simulink library "vmc"  (R2021b)
settings: Solver=VariableStepAuto  StartTime=0.0  StopTime=10.0  RelTol=1e-3
undefined symbols (not defined in the file): AVMC_ACCDeltaTqGradeGn_X_deg, AVMC_ACCDeltaTqIGain4OVRD_X_kph, AVMC_ACCDeltaTqIGain4OVRD_Y_mps2, AVMC_ACCDeltaTqIGain_X_kph, AVMC_ACCDeltaTqIGain_Y_mps2, AVMC_ACCDeltaTqPGain_X_kph, AVMC_ACCDeltaTqPGain_Y_kph, AVMC_ACCGradeofst_X_G, AVMC_ACCGradeofst_Y_pct, AVMC_ACCLoSpdTqLoLim4JP_X_kph, AVMC_ACCLoSpdTqLoLim4JP_Y_deg, AVMC_ACCLoSpdTqLowerLim_X_kph, AVMC_ACCLoSpdTqLowerLim_Y_deg, AVMC_ACCReqAccelGain_X_mps2, AVMC_ACCReqAccelGain_Y_enum, AVMC_ADSPosGFBDeltaTq_X_kph, AVMC_ADSPosGFBDeltaTq_Y_mps2, AVMC_AggressJerkPCT4AT_X_kph, AVMC_AggressJerkPCT_X_kph, AVMC_AggressLimitPCT4AT_X_kph, AVMC_AggressLimitPCT_X_kph, AVMC_DECGradeofst_X_G, AVMC_DECGradeofst_Y_pct, AVMC_DISCDeltaTqIGain_X_kph, AVMC_DISCDeltaTqIGain_Y_mps2, AVMC_DISCDeltaTqPGain_X_kph, AVMC_DISCDeltaTqPGain_Y_kph, AVMC_EPSForceSelect_X_enum, AVMC_EPSForceSelect_Y_enum, AVMC_EPSForceSelectD21_X_enum, AVMC_EPSForceSelectD21_Y_enum, AVMC_ESCRegenOut_X_kph, AVMC_ESCRegenOut_Y_Deg, AVMC_ESCRegenOutEnSpd_X_Deg, AVMC_EstPitchSlopeTs_X_kph, AVMC_GradeCompFlt_X_kph, AVMC_GyroYBandLo_X_Gps, AVMC_HoldResTq_X_kph, AVMC_ISOAccLimit_X_mps, AVMC_ISODecLimit_X_mps, AVMC_ISOJerk_X_mps, AVMC_LatESCRegenOut_X_kph, AVMC_LatESCRegenOut_Y_Deg, AVMC_LongAccDeadZone_X_kph, AVMC_LongAccFiltTsforP2_X_Gps, AVMC_MCPresBaseTq_X_bar, AVMC_MSAPedalOvrd_X_kph, AVMC_MSASpdBand_X_kph, AVMC_MSATqDownEndTq_X_kph, AVMC_MSATqDownTime_X_kph, AVMC_NegZCHoldTq_X_kph, AVMC_OPDDisSlideRate_X_Deg, AVMC_OVRD2ActSR2FCMCMD_X_mps2, AVMC_PedalTqRWhlRatio_X_Nm, AVMC_PedalTqRWhlRatio_Y_gps, AVMC_PedalTqRWhlSlipGain_X_rat, AVMC_PedalTqRWhlSlipGain_Y_kph, AVMC_PedalTqRWhSTRGGain_X_deg, AVMC_PedalTqRWhSTRGGain_Y_kph, AVMC_PosZCHoldTq_X_kph ... (+593)
libraries: hcu_lib x143, simulink x96, tqr x4, $bdroot x1, simulink_extras x1
(part 15 of 17)

== system vmc/VMC/VMC/Long Acceleration Calculation/Estimate Slope1/SR_Latch1 ==
  set : Inport
  reset : Inport  Port=2
  Data Type Conversion : DataTypeConversion  OutDataTypeStr=boolean
  Logical Operator : Logic  AllPortsSameDT=off  OutDataTypeStr=boolean
  Logical Operator1 : Logic  Operator=NOT  AllPortsSameDT=off  OutDataTypeStr=boolean
  Switch1 : Switch  Criteria=u2 ~= 0  Threshold=0.5
      settings: AttributesFormatString=<Criteria=%<Criteria>>
  Switch2 : Switch  Criteria=u2 ~= 0  Threshold=0.5
      settings: AttributesFormatString=<Criteria=%<Criteria>>
  Unit Delay : UnitDelay  SampleTime=-1  HasFrameUpgradeWarning=on
  latched : Outport
  wires:
  Data Type Conversion/1 -> Unit Delay/1, latched/1
  Switch1/1 -> Data Type Conversion/1
  set/1 -> Switch1/1, Logical Operator/1
  reset/1 -> Switch2/2, Logical Operator1/1
  Unit Delay/1 -> Switch2/3
  Switch2/1 -> Switch1/3
  Logical Operator/1 -> Switch1/2
  Logical Operator1/1 -> Logical Operator/2, Switch2/1

== system vmc/VMC/VMC/Long Acceleration Calculation/Estimate Slope1/SR_Latch2 ==
  set : Inport
  reset : Inport  Port=2
  Data Type Conversion : DataTypeConversion  OutDataTypeStr=boolean
  Logical Operator : Logic  AllPortsSameDT=off  OutDataTypeStr=boolean
  Logical Operator1 : Logic  Operator=NOT  AllPortsSameDT=off  OutDataTypeStr=boolean
  Switch1 : Switch  Criteria=u2 ~= 0  Threshold=0.5
      settings: AttributesFormatString=<Criteria=%<Criteria>>
  Switch2 : Switch  Criteria=u2 ~= 0  Threshold=0.5
      settings: AttributesFormatString=<Criteria=%<Criteria>>
  Unit Delay : UnitDelay  SampleTime=-1  HasFrameUpgradeWarning=on
  latched : Outport
  wires:
  Logical Operator1/1 -> Switch2/1, Logical Operator/2
  Logical Operator/1 -> Switch1/2
  Switch2/1 -> Switch1/3
  Unit Delay/1 -> Switch2/3
  reset/1 -> Logical Operator1/1, Switch2/2
  set/1 -> Logical Operator/1, Switch1/1
  Switch1/1 -> Data Type Conversion/1
  Data Type Conversion/1 -> latched/1, Unit Delay/1

== system vmc/VMC/VMC/Long Acceleration Calculation/Estimate Slope1/SR_Latch3 ==
  set : Inport
  reset : Inport  Port=2
  Data Type Conversion : DataTypeConversion  OutDataTypeStr=boolean
  Logical Operator : Logic  AllPortsSameDT=off  OutDataTypeStr=boolean
  Logical Operator1 : Logic  Operator=NOT  AllPortsSameDT=off  OutDataTypeStr=boolean
  Switch1 : Switch  Criteria=u2 ~= 0  Threshold=0.5
      settings: AttributesFormatString=<Criteria=%<Criteria>>
  Switch2 : Switch  Criteria=u2 ~= 0  Threshold=0.5
      settings: AttributesFormatString=<Criteria=%<Criteria>>
  Unit Delay : UnitDelay  SampleTime=-1  HasFrameUpgradeWarning=on
  latched : Outport
  wires:
  Logical Operator1/1 -> Switch2/1, Logical Operator/2
  Logical Operator/1 -> Switch1/2
  Switch2/1 -> Switch1/3
  Unit Delay/1 -> Switch2/3
  reset/1 -> Logical Operator1/1, Switch2/2
  set/1 -> Logical Operator/1, Switch1/1
  Switch1/1 -> Data Type Conversion/1
  Data Type Conversion/1 -> latched/1, Unit Delay/1

== system vmc/VMC/VMC/Long Acceleration Calculation/Estimate Slope1/SR_Latch6 ==
  set : Inport
  reset : Inport  Port=2
  Data Type Conversion : DataTypeConversion  OutDataTypeStr=boolean
  Logical Operator : Logic  AllPortsSameDT=off  OutDataTypeStr=boolean
  Logical Operator1 : Logic  Operator=NOT  AllPortsSameDT=off  OutDataTypeStr=boolean
  Switch1 : Switch  Criteria=u2 ~= 0  Threshold=0.5
      settings: AttributesFormatString=<Criteria=%<Criteria>>
  Switch2 : Switch  Criteria=u2 ~= 0  Threshold=0.5
      settings: AttributesFormatString=<Criteria=%<Criteria>>
  Unit Delay : UnitDelay  SampleTime=-1  HasFrameUpgradeWarning=on
  latched : Outport
  wires:
  Logical Operator1/1 -> Switch2/1, Logical Operator/2
  Logical Operator/1 -> Switch1/2
  Switch2/1 -> Switch1/3
  Unit Delay/1 -> Switch2/3
  reset/1 -> Logical Operator1/1, Switch2/2
  set/1 -> Logical Operator/1, Switch1/1
  Switch1/1 -> Data Type Conversion/1
  Data Type Conversion/1 -> latched/1, Unit Delay/1

== system vmc/VMC/VMC/Long Acceleration Calculation/Estimate Slope1/Triggered Subsystem ==
  In1 : Inport
  Trigger : TriggerPort  VariantControl=(inherit)
  Out1 : Outport
  wires:
  In1/1 -> Out1/1

== system vmc/VMC/VMC/MSA function/MSADemandTorqueCalculation/Triggered Subsystem ==
  In1 : Inport
  Trigger : TriggerPort  VariantControl=(inherit)
  Out1 : Outport
  wires:
  In1/1 -> Out1/1

== system vmc/VMC/VMC/MSA function/MSATorqueSourceDetermination/Triggered Subsystem2 ==
  In1 : Inport
  Trigger : TriggerPort  VariantControl=(inherit)
  Out1 : Outport
  wires:
  In1/1 -> Out1/1

== system vmc/VMC/VMC/SPD2ACC/Required_Acceleration/Triggered Subsystem ==
  In1 : Inport
  In2 : Inport  Port=2
  Trigger : TriggerPort  VariantControl=(inherit)
  Add29 : Sum  Inputs=+-
  Constant216 : Constant  Value=KVMC_ReqBrkInDecSRTime_s
  Divide : Product  Inputs=*/
  Out1 : Outport
  wires:
  In1/1 -> Add29/2
  In2/1 -> Add29/1
  Add29/1 -> Divide/1
  Constant216/1 -> Divide/2
  Divide/1 -> Out1/1

== system vmc/VMC/VMC/SPD2ACC/Required_Acceleration/Triggered Subsystem4 ==
  In1 : Inport
  Trigger : TriggerPort  VariantControl=(inherit)
  Out1 : Outport
  wires:
  In1/1 -> Out1/1

== system vmc/VMC/VMC/SPD2ACC/Required_Acceleration/Triggered Subsystem6 ==
  In1 : Inport
  In2 : Inport  Port=2
  In3 : Inport  Port=3
  Trigger : TriggerPort  VariantControl=(inherit)
  Out1 : Outport
  Out2 : Outport  Port=2
  Out3 : Outport  Port=3
  wires:
  In3/1 -> Out3/1
  In2/1 -> Out2/1
  In1/1 -> Out1/1

== system vmc/VMC/VMC/SPD2ACC/Required_Acceleration/Triggered Subsystem7 ==
  In1 : Inport
  Trigger : TriggerPort  VariantControl=(inherit)
  Out1 : Outport
  wires:
  In1/1 -> Out1/1

== system vmc/VMC/VMC/SafetyControl/LongAccel_EstSlope_FrontRearSlipSpd/Estimate Slope ==
  VINP_LongAccel_Gps : Inport
  VVMC_VehicleSpeed_kph : Inport  Port=2
  VINP_GRADE_deg : Inport  Port=3
  task_time_s : Inport  Port=4
  Add : Sum  Inputs=+-
  Asin : Trigonometry  Operator=asin
  Constant : Constant  Tag=struct('comment',struct('text','','placement',1),'output',struct('width',1,'name','$S_$B','unit','','type','Int16','offset',0,'max',NaN,'min',NaN,'freeze',1,'lsb',1,'arb',0,'class','default','address','','description','','value','0','tolerance',1,'show',0),'date',731450.689904282)  Value=ZERO_FLOAT  OutDataTypeStr=single
  Constant1 : Constant  Value=KVMC_EstSlopeLongAccelTs_c
  Constant2 : Constant  Value=KVMC_EstSlopeVehSpdTs_c
  Constant28 : Constant  Value=MINUSONE_FLOAT
  Constant29 : Constant  Value=ONE_FLOAT
  Constant3 : Constant  Value=KVMC_EstSlopeTs_c
  Constant4 : Constant  Value=KVMC_EstSlopeSW_flg
  Constant5 : Constant  Tag=struct('comment',struct('text','','placement',1),'output',struct('width',1,'name','$S_$B','unit','','type','Int16','offset',0,'max',NaN,'min',NaN,'freeze',1,'lsb',1,'arb',0,'class','default','address','','description','','value','2','tolerance',1,'show',0),'date',731450.690075)  Value=TRUE
  FirstOrderFilter : hcu_lib/Basic_Blocks/FirstOrderFilter
  FirstOrderFilter1 : hcu_lib/Basic_Blocks/FirstOrderFilter
  FirstOrderFilter2 : hcu_lib/Basic_Blocks/FirstOrderFilter
  Gain : Gain  Gain=KPH2MPS
  Gain1 : Gain  Gain=1/GRAVITY_G
  Gain2 : Gain  Gain=RAD2DEG
  Product : Product  Tag=struct('comment',struct('text','','placement',1),'logdata',struct('maxnumvals',inf,'plotchannels',[],'stepsize',0,'downsampling',1,'loggingmode',3,'channels',1),'output',struct('width',1,'name','$S_$B','unit','','type','Int32Bin15','offset',0,'max',65535,'min',-65536,'freeze',1,'lsb',2^-15,'arb',0,'class','default','address','','description','','autoscalingmode',1,'lowerheadroom',1,'upperheadroom',1,'headroomunit','bit','checkmin',0,'checkmax',0,'show',0),'inputs','*/','exceptionhandling',1,'date',731458.438505301)  Inputs=*/  InputSameDT=on  RndMeth=Zero  SaturateOnIntegerOverflow=on  OutDataTypeStr=Inherit: Same as first input
  Saturation Dynamic3 : simulink/Discontinuities/Saturation Dynamic  OutMin=[]  OutMax=[]  OutDataTypeStr=Inherit: Same as second input  OutDataType=fixdt(1, 16)  OutScaling=2^-10  DoSatur=off
  Sum : Sum  Tag=struct('comment',struct('text','','placement',1),'logdata',struct('maxnumvals',inf,'plotchannels',[],'stepsize',0,'downsampling',1,'loggingmode',3,'channels',1),'output',struct('width',1,'name','$S_$B','unit','','type','Int32Bin15','offset',0,'max',65535,'min',-65536,'freeze',1,'lsb',2^-15,'arb',0,'class','default','address','','description','','autoscalingmode',1,'lowerheadroom',1,'upperheadroom',1,'headroomunit','bit','checkmin',0,'checkmax',0,'show',0),'inputs','+-','date',731450.688943275)  Inputs=+-  InputSameDT=on  SaturateOnIntegerOverflow=on  OutDataTypeStr=Inherit: Same as first input
  Switch : Switch  Criteria=u2 > Threshold
  Switch1 : Switch  Tag=struct('comment',struct('text','','placement',1),'logdata',struct('maxnumvals',inf,'plotchannels',[],'stepsize',0,'downsampling',1,'loggingmode',3,'channels',1),'output',struct('width',1,'name','$S_$B','unit','','type','Int32Bin15','offset',0,'max',65535,'min',-65536,'freeze',1,'lsb',2^-15,'arb',0,'class','default','address','','description','','autoscalingmode',1,'lowerheadroom',1,'upperheadroom',1,'headroomunit','bit','checkmin',0,'checkmax',0,'show',0),'threshold',struct('width',1,'name','$S_$B_threshold','unit','','type','Int16','offset',0,'max',NaN,'min',NaN,'freeze',1,'lsb',1,'arb',0,'class','default','address','','description','','value','1','scalar',0),'date',731458.438569977)  Criteria=u2 > Threshold  SaturateOnIntegerOverflow=on  InputSameDT=on
  UnitDelay1 : UnitDelay  Tag=struct('comment',struct('text','','placement',1),'logdata',struct('maxnumvals',inf,'plotchannels',[],'stepsize',0,'downsampling',1,'loggingmode',3,'channels',1),'output',struct('width',1,'name','$S_$B','unit','','type','Int32Bin15','offset',0,'max',65535,'min',-65536,'freeze',1,'lsb',2^-15,'arb',0,'class','default','address','','description','','autoscalingmode',1,'lowerheadroom',1,'upperheadroom',1,'headroomunit','bit','checkmin',0,'checkmax',0,'show',0,'initial','0'),'state',0,'dt','-1','date',731450.687911019)  SampleTime=-1  HasFrameUpgradeWarning=on
  UnitDelay2 : UnitDelay  Tag=struct('comment',struct('text','','placement',1),'logdata',struct('maxnumvals',inf,'plotchannels',[],'stepsize',0,'downsampling',1,'loggingmode',3,'channels',1),'output',struct('width',1,'name','$S_$B','unit','','type','UInt8','offset',0,'max',255,'min',0,'freeze',1,'lsb',1,'arb',0,'class','default','address','','description','','autoscalingmode',1,'lowerheadroom',1,'upperheadroom',1,'headroomunit','bit','checkmin',0,'checkmax',0,'show',0,'initial','0'),'state',0,'dt','-1','date',731450.690382801)  InitialCondition=FALSE  SampleTime=-1  StateName=first_pass  HasFrameUpgradeWarning=on
  VVMC_EstSlopeCal_Deg : Outport
  wires:
  VINP_GRADE_deg/1 -> Switch/3
  Constant4/1 -> Switch/2
  [task_time_s] -> FirstOrderFilter1/2
  Constant2/1 -> FirstOrderFilter1/3
  Constant3/1 -> FirstOrderFilter2/3
  [task_time_s] -> FirstOrderFilter2/2
  Constant1/1 -> FirstOrderFilter/3
  [task_time_s] -> FirstOrderFilter/2
  Switch/1 -> VVMC_EstSlopeCal_Deg/1  "VVMC_EstSlopeCal_Deg"
  FirstOrderFilter2/1 -> Switch/1
  Gain2/1 -> FirstOrderFilter2/1
  Asin/1 -> Gain2/1
  Product/1 -> Gain1/1
  FirstOrderFilter1/1 -> Gain/1
  FirstOrderFilter/1 -> Add/1
  Add/1 -> Saturation Dynamic3/2  "sum"
  Gain1/1 -> Add/2
  VINP_LongAccel_Gps/1 -> FirstOrderFilter/1
  VVMC_VehicleSpeed_kph/1 -> FirstOrderFilter1/1
  task_time_s/1 -> [task_time_s]
  Constant/1 -> Switch1/3
  UnitDelay2/1 -> Switch1/2
  Constant5/1 -> UnitDelay2/1
  [task_time_s] -> Product/2
  UnitDelay1/1 -> Sum/2
  Gain/1 -> Sum/1, UnitDelay1/1
  Sum/1 -> Switch1/1
  Switch1/1 -> Product/1
  Constant28/1 -> Saturation Dynamic3/3
  Constant29/1 -> Saturation Dynamic3/1
  Saturation Dynamic3/1 -> Asin/1

== system vmc/VMC/VMC/SafetyControl/SafetyControlJudgement/FrontRearSlipRatio ==
  VVMC_LFWhlSpeedRollAve_kph : Inport
  VVMC_RFWhlSpeedRollAve_kph : Inport  Port=2
  VVMC_LRWhlSpeedRollAve_kph : Inport  Port=3
  VVMC_RRWhlSpeedRollAve_kph : Inport  Port=4
  VINP_LFRawWhlSpeedV_flg : Inport  Port=5
  VINP_RFRawWhlSpeedV_flg : Inport  Port=6
  VINP_LRRawWhlSpeedV_flg : Inport  Port=7
  VINP_RRRawWhlSpeedV_flg : Inport  Port=8
  Constant : Constant  Value=KVMC_FrontRearSlipRatioTHR_kph
  Constant1 : Constant  Value=TRUE
  Constant2 : Constant  Value=FALSE
  Constant3 : Constant  Value=TWO_FLOAT
  Constant4 : Constant  Value=ZERO_FLOAT
  FrontRearSlipRatioJudgement : Stateflow chart  TreatAsAtomicUnit=on
  "VVMC_FrontRearSlipRatioCtrl_flg " : Outport
  wires:
  VVMC_LFWhlSpeedRollAve_kph/1 -> [VVMC_LFWhlSpeedRollAve_kph]
  VVMC_RFWhlSpeedRollAve_kph/1 -> [VVMC_RFWhlSpeedRollAve_kph]
  VVMC_LRWhlSpeedRollAve_kph/1 -> [VVMC_LRWhlSpeedRollAve_kph]
  VVMC_RRWhlSpeedRollAve_kph/1 -> [VVMC_RRWhlSpeedRollAve_kph]
  VINP_LFRawWhlSpeedV_flg/1 -> [VINP_LFRawWhlSpeedV_flg]
  VINP_RFRawWhlSpeedV_flg/1 -> [VINP_RFRawWhlSpeedV_flg]
  VINP_LRRawWhlSpeedV_flg/1 -> [VINP_LRRawWhlSpeedV_flg]
  VINP_RRRawWhlSpeedV_flg/1 -> [VINP_RRRawWhlSpeedV_flg]
  [VINP_LRRawWhlSpeedV_flg] -> FrontRearSlipRatioJudgement/7(VINP_LRRawWhlSpeedV_flg)
  [VINP_LFRawWhlSpeedV_flg] -> FrontRearSlipRatioJudgement/5(VINP_LFRawWhlSpeedV_flg)
  [VVMC_LRWhlSpeedRollAve_kph] -> FrontRearSlipRatioJudgement/3(VVMC_LRWhlSpeedRollAve_kph)
  [VINP_RFRawWhlSpeedV_flg] -> FrontRearSlipRatioJudgement/6(VINP_RFRawWhlSpeedV_flg)
  [VVMC_LFWhlSpeedRollAve_kph] -> FrontRearSlipRatioJudgement/1(VVMC_LFWhlSpeedRollAve_kph)
  [VVMC_RFWhlSpeedRollAve_kph] -> FrontRearSlipRatioJudgement/2(VVMC_RFWhlSpeedRollAve_kph)
  [VVMC_RRWhlSpeedRollAve_kph] -> FrontRearSlipRatioJudgement/4(VVMC_RRWhlSpeedRollAve_kph)
  [VINP_RRRawWhlSpeedV_flg] -> FrontRearSlipRatioJudgement/8(VINP_RRRawWhlSpeedV_flg)
  Constant/1 -> FrontRearSlipRatioJudgement/9(KVMC_FrontRearSlipRatioTHR_kph)
  Constant1/1 -> FrontRearSlipRatioJudgement/10(TRUE)
  FrontRearSlipRatioJudgement/1(VVMC_FrontRearSlipRatioCtrl_flg) -> [VVMC_FrontRearSlipRatioCtrl_flg]
  [VVMC_FrontRearSlipRatioCtrl_flg] -> "VVMC_FrontRearSlipRatioCtrl_flg "/1
  Constant2/1 -> FrontRearSlipRatioJudgement/11(FALSE)
  Constant3/1 -> FrontRearSlipRatioJudgement/12(TWO_FLOAT)
  Constant4/1 -> FrontRearSlipRatioJudgement/13(ZERO_FLOAT)

== system vmc/VMC/VMC/SafetyControl/SafetyControlJudgement/LateralAccelerationControl ==
  VVMC_LatAccRollAve_Gps : Inport
  VINP_LatAccelV_flg : Inport  Port=2
  Abs : Abs
  Constant : Constant  Value=KVMC_LatAccCtrlTHR_Gps
  Logical Operator : Logic  Operator=OR  AllPortsSameDT=off  OutDataTypeStr=boolean
  Relational Operator : RelationalOperator  OutDataTypeStr=boolean  RndMeth=Simplest
  VVMC_LatAccCtrl_flg : Outport
  wires:
  VVMC_LatAccRollAve_Gps/1 -> [VVMC_LatAccRollAve_Gps]
  VINP_LatAccelV_flg/1 -> [VINP_LatAccelV_flg]
  [VVMC_LatAccCtrl_flg] -> VVMC_LatAccCtrl_flg/1
  [VVMC_LatAccRollAve_Gps] -> Abs/1
  Constant/1 -> Relational Operator/2
  Relational Operator/1 -> Logical Operator/1
  [VINP_LatAccelV_flg] -> Logical Operator/2
  Logical Operator/1 -> [VVMC_LatAccCtrl_flg]  "VVMC_LatAccCtrl_flg"
  Abs/1 -> Relational Operator/1

== system vmc/VMC/VMC/SafetyControl/SafetyControlJudgement/RearWheelSlipRatio ==
  VVMC_LRWhlSpeedRollAve_kph : Inport
  VVMC_RRWhlSpeedRollAve_kph : Inport  Port=2
  VINP_LRRawWhlSpeedV_flg : Inport  Port=3
  VINP_RRRawWhlSpeedV_flg : Inport  Port=4
  Constant : Constant  Value=KVMC_RearWhlSlipRatioTHR_kph
  Constant1 : Constant  Value=TRUE
  Constant2 : Constant  Value=FALSE
  FrontRearSlipRatioJudgement : Stateflow chart  TreatAsAtomicUnit=on
  "VVMC_RearWhlSlipRatioCtrl_flg " : Outport
  wires:
  Constant2/1 -> FrontRearSlipRatioJudgement/7(FALSE)
  [VVMC_RearWhlSlipRatioCtrl_flg] -> "VVMC_RearWhlSlipRatioCtrl_flg "/1
  FrontRearSlipRatioJudgement/1(VVMC_RearWhlSlipRatioCtrl_flg) -> [VVMC_RearWhlSlipRatioCtrl_flg]
  Constant1/1 -> FrontRearSlipRatioJudgement/6(TRUE)
  Constant/1 -> FrontRearSlipRatioJudgement/5(KVMC_RearWhlSlipRatioTHR_kph)
  [VINP_RRRawWhlSpeedV_flg] -> FrontRearSlipRatioJudgement/4(VINP_RRRawWhlSpeedV_flg)
  [VVMC_RRWhlSpeedRollAve_kph] -> FrontRearSlipRatioJudgement/2(VVMC_RRWhlSpeedRollAve_kph)
  [VVMC_LRWhlSpeedRollAve_kph] -> FrontRearSlipRatioJudgement/1(VVMC_LRWhlSpeedRollAve_kph)
  [VINP_LRRawWhlSpeedV_flg] -> FrontRearSlipRatioJudgement/3(VINP_LRRawWhlSpeedV_flg)
  VINP_RRRawWhlSpeedV_flg/1 -> [VINP_RRRawWhlSpeedV_flg]
  VINP_LRRawWhlSpeedV_flg/1 -> [VINP_LRRawWhlSpeedV_flg]
  VVMC_RRWhlSpeedRollAve_kph/1 -> [VVMC_RRWhlSpeedRollAve_kph]
  VVMC_LRWhlSpeedRollAve_kph/1 -> [VVMC_LRWhlSpeedRollAve_kph]

== system vmc/VMC/VMC/SafetyControl/SafetyControlJudgement/SafetyControlJudgement ==
  VVMC_FrontRearSlipRatioCtrl_flg : Inport
  VVMC_RearWhlSlipRatioCtrl_flg : Inport  Port=2
  VVMC_SingleWhlSlipRatioCtrl_flg : Inport  Port=3
  VVMC_LatAccCtrl_flg : Inport  Port=4
  VVMC_FeatArbitrFinal_enum : Inport  Port=5
  AND : Logic  AllPortsSameDT=off  OutDataTypeStr=boolean
  Constant1 : Constant  Value=KVMC_SafetyCtrlForACCSW_flg
  Constant17 : Constant  Value=ENUM_FEATARBITRSTA_DISC
  Constant2 : Constant  Value=ENUM_FEATARBITRSTA_ACC
  Logical Operator : Logic  Operator=OR  Inputs=4  AllPortsSameDT=off  OutDataTypeStr=boolean
  Logical Operator1 : Logic  AllPortsSameDT=off  OutDataTypeStr=boolean
  OR : Logic  Operator=OR  AllPortsSameDT=off  OutDataTypeStr=boolean
  Relational Operator : RelationalOperator  Operator===  OutDataTypeStr=boolean  RndMeth=Simplest
  Relational Operator1 : RelationalOperator  Operator===  OutDataTypeStr=boolean  RndMeth=Simplest
  "VVMC_SafetyCtrl_flg " : Outport
  wires:
  OR/1 -> Logical Operator1/2
  AND/1 -> OR/2
  Constant1/1 -> AND/2
  Relational Operator1/1 -> AND/1
  [VVMC_FeatArbitrFinal_enum] -> Relational Operator1/1
  Constant2/1 -> Relational Operator1/2
  VVMC_FrontRearSlipRatioCtrl_flg/1 -> [VVMC_FrontRearSlipRatioCtrl_flg]
  VVMC_RearWhlSlipRatioCtrl_flg/1 -> [VVMC_RearWhlSlipRatioCtrl_flg]
  VVMC_SingleWhlSlipRatioCtrl_flg/1 -> [VVMC_SingleWhlSlipRatioCtrl_flg]
  [VVMC_SafetyCtrl_flg] -> "VVMC_SafetyCtrl_flg "/1
  [VVMC_FrontRearSlipRatioCtrl_flg] -> Logical Operator/1
  [VVMC_RearWhlSlipRatioCtrl_flg] -> Logical Operator/2
  [VVMC_SingleWhlSlipRatioCtrl_flg] -> Logical Operator/3
  Logical Operator1/1 -> [VVMC_SafetyCtrl_flg]
  VVMC_LatAccCtrl_flg/1 -> [VVMC_LatAccCtrl_flg]
  [VVMC_LatAccCtrl_flg] -> Logical Operator/4
  VVMC_FeatArbitrFinal_enum/1 -> [VVMC_FeatArbitrFinal_enum]
  Constant17/1 -> Relational Operator/2
  Logical Operator/1 -> Logical Operator1/1
  Relational Operator/1 -> OR/1
  [VVMC_FeatArbitrFinal_enum] -> Relational Operator/1

== system vmc/VMC/VMC/SafetyControl/SafetyControlJudgement/SingleWheelSlipRatio ==
  VVMC_VehicleSpeed_kph : Inport
  VVMC_LFWhlSpeedRollAve_kph : Inport  Port=2
  VVMC_RFWhlSpeedRollAve_kph : Inport  Port=3
  VVMC_LRWhlSpeedRollAve_kph : Inport  Port=4
  VVMC_RRWhlSpeedRollAve_kph : Inport  Port=5
  VINP_LFRawWhlSpeedV_flg : Inport  Port=6
  VINP_RFRawWhlSpeedV_flg : Inport  Port=7
  VINP_LRRawWhlSpeedV_flg : Inport  Port=8
  VINP_RRRawWhlSpeedV_flg : Inport  Port=9
  Constant : Constant  Value=KVMC_SingleWhlSlipRatioTHR_kph
  Constant1 : Constant  Value=TRUE
  Constant2 : Constant  Value=FALSE
  SingleWheelSlipRatioJudgement : Stateflow chart  TreatAsAtomicUnit=on
  VVMC_SingleWhlSlipRatioCtrl_flg : Outport
  wires:
  Constant2/1 -> SingleWheelSlipRatioJudgement/12(FALSE)
  [VVMC_SingleWhlSlipRatioCtrl_flg] -> VVMC_SingleWhlSlipRatioCtrl_flg/1
  SingleWheelSlipRatioJudgement/1(VVMC_SingleWhlSlipRatioCtrl_flg) -> [VVMC_SingleWhlSlipRatioCtrl_flg]
  Constant1/1 -> SingleWheelSlipRatioJudgement/11(TRUE)
  Constant/1 -> SingleWheelSlipRatioJudgement/10(KVMC_SingleWhlSlipRatioTHR_kph)
  [VINP_RRRawWhlSpeedV_flg] -> SingleWheelSlipRatioJudgement/9(VINP_RRRawWhlSpeedV_flg)
  [VVMC_RRWhlSpeedRollAve_kph] -> SingleWheelSlipRatioJudgement/5(VVMC_RRWhlSpeedRollAve_kph)
  [VVMC_RFWhlSpeedRollAve_kph] -> SingleWheelSlipRatioJudgement/3(VVMC_RFWhlSpeedRollAve_kph)
  [VVMC_LFWhlSpeedRollAve_kph] -> SingleWheelSlipRatioJudgement/2(VVMC_LFWhlSpeedRollAve_kph)
  [VINP_RFRawWhlSpeedV_flg] -> SingleWheelSlipRatioJudgement/7(VINP_RFRawWhlSpeedV_flg)
  [VVMC_LRWhlSpeedRollAve_kph] -> SingleWheelSlipRatioJudgement/4(VVMC_LRWhlSpeedRollAve_kph)
  [VINP_LFRawWhlSpeedV_flg] -> SingleWheelSlipRatioJudgement/6(VINP_LFRawWhlSpeedV_flg)
  [VINP_LRRawWhlSpeedV_flg] -> SingleWheelSlipRatioJudgement/8(VINP_LRRawWhlSpeedV_flg)
  VINP_RRRawWhlSpeedV_flg/1 -> [VINP_RRRawWhlSpeedV_flg]
  VINP_LRRawWhlSpeedV_flg/1 -> [VINP_LRRawWhlSpeedV_flg]
  VINP_RFRawWhlSpeedV_flg/1 -> [VINP_RFRawWhlSpeedV_flg]
  VINP_LFRawWhlSpeedV_flg/1 -> [VINP_LFRawWhlSpeedV_flg]
  VVMC_RRWhlSpeedRollAve_kph/1 -> [VVMC_RRWhlSpeedRollAve_kph]
  VVMC_LRWhlSpeedRollAve_kph/1 -> [VVMC_LRWhlSpeedRollAve_kph]
  VVMC_RFWhlSpeedRollAve_kph/1 -> [VVMC_RFWhlSpeedRollAve_kph]
  VVMC_LFWhlSpeedRollAve_kph/1 -> [VVMC_LFWhlSpeedRollAve_kph]
  VVMC_VehicleSpeed_kph/1 -> [VVMC_VehicleSpeed_kph]
  [VVMC_VehicleSpeed_kph] -> SingleWheelSlipRatioJudgement/1(VVMC_VehicleSpeed_kph)

== system vmc/VMC/VMC/Slide Rate  Calculation/4Wheel Calculation/Determination ==
  VVMC_4WheelLongAcc_Gps : Inport
  task_time_s : Inport  Port=2
  VVMC_VehicleSpeed_kph : Inport  Port=3
  VTQD_GearActualPosn_enum : Inport  Port=4
  VVMC_LFWhlSkid_flg : Inport  Port=5
  VVMC_RFWhlSkid_flg : Inport  Port=6
  VVMC_LRWhlSkid_flg : Inport  Port=7
  VVMC_RRWhlSkid_flg : Inport  Port=8
  VVMC_LF4WhlSpdSlideRate_pct : Inport  Port=9
  VVMC_RF4WhlSpdSlideRate_pct : Inport  Port=10
  VVMC_LR4WhlSpdSlideRate_pct : Inport  Port=11
  VVMC_RR4WhlSpdSlideRate_pct : Inport  Port=12
  VTQD_AfterAvailableTqDemFr_Nm : Inport  Port=13
  VTQD_AfterAvailableTqDemRr_Nm : Inport  Port=14
  VVMC_LFPreVehSpd_kph : Inport  Port=15
  VVMC_RFPreVehSpd_kph : Inport  Port=16
  VVMC_LRPreVehSpd_kph : Inport  Port=17
  VVMC_RRPreVehSpd_kph : Inport  Port=18
  AND : Logic  Inputs=4  AllPortsSameDT=off  OutDataTypeStr=boolean
  Add : Sum
  Add1 : Sum  Inputs=++++
  Add17 : Sum
  Add2 : Sum
  Constant1 : Constant  Value=GRAVITY_G
  Constant10 : Constant  Value=3
  Constant11 : Constant  Value=KPH2MPS
  Constant2 : Constant  Value=MPS2KPH
  Constant3 : Constant  Value=KVMC_PreVehSpdNum_c
  Constant4 : Constant  Value=ZERO_FLOAT
  Constant44 : Constant  Value=KPH2MPS
  Constant45 : Constant  Value=ZERO_FLOAT
  Constant46 : Constant  Value=ENUM_GEARACTUALPOSN_D
  Constant47 : Constant  Value=ENUM_GEARACTUALPOSN_R
  Constant48 : Constant  Value=KVMC_PreVehSpdCalSW_flg
  Constant5 : Constant  Value=KVMC_PreVehSpdSource_enum
  Constant6 : Constant
  Constant7 : Constant  Value=KVMC_PreVehSpdSource_enum
  Constant8 : Constant  Value=2
  Constant9 : Constant  Value=KVMC_PreVehSpdSource_enum
  Delay : Delay  DelayLength=1
  Delay5 : Delay  DelayLength=1
  Divide : Product  Inputs=*/
  Equal{,1..4} (5 alike) : RelationalOperator  Operator===  OutDataTypeStr=boolean  RndMeth=Simplest
  Max : MinMax  Function=max  Inputs=4
  Max1 : MinMax  Inputs=4
  Max2 : MinMax  Function=max  Inputs=4
  Max3 : MinMax  Inputs=4
  OR : Logic  Operator=OR  AllPortsSameDT=off  OutDataTypeStr=boolean
  OR1 : Logic  Operator=OR  AllPortsSameDT=off  OutDataTypeStr=boolean
  Product : Product
  Product1 : Product  Inputs=3
  Product2 : Product
  Product3 : Product
  Relational Operator1 : RelationalOperator  Operator=<=  OutDataTypeStr=boolean  RndMeth=Simplest
  Relational Operator16 : RelationalOperator  Operator=<=  OutDataTypeStr=boolean  RndMeth=Simplest
  Saturation : Saturate  UpperLimit=KVMC_PredVehSpdLimit_mps  LowerLimit=ZERO_FLOAT
  Switch{,1..4,9..10} (7 alike) : Switch  Criteria=u2 > Threshold
  VVMC_PredictVehSpd_kph : Outport
  VVMC_AllWhlSkid_flg : Outport  Port=2
  VVMC_4WhlSpdSlideRate_pct : Outport  Port=3
  wires:
  [VVMC_Min4WhlPreVehSpd_kph] -> Switch1/3
  [VVMC_Max4WhlPreVehSpd_kph] -> Switch1/1
  [VTQD_AfterAvailableTqDemRr_Nm] -> Add2/2
  [VTQD_AfterAvailableTqDemFr_Nm] -> Add2/1
  Switch4/1 -> [VVMC_PredictVehSpd_kph]  "VVMC_PredictVehSpd_kph"
  [VVMC_PredictVehSpd3_kph] -> Switch4/1
  Equal4/1 -> Switch4/2
  Constant10/1 -> Equal4/2
  Constant9/1 -> Equal4/1
  Switch3/1 -> Switch4/3
  [VVMC_PredictVehSpd2_kph] -> Switch3/1
  Switch2/1 -> Switch3/3
  Constant7/1 -> Equal3/1
  Constant8/1 -> Equal3/2
  Equal3/1 -> Switch3/2
  [VVMC_VehicleSpeed_kph] -> Switch2/3
  [VVMC_PredictVehSpd1_kph] -> Switch2/1
  Equal2/1 -> Switch2/2
  Constant6/1 -> Equal2/2
  Constant5/1 -> Equal2/1
  [VVMC_PredictVehSpd1_kph] -> Delay5/1
  Switch1/1 -> [VVMC_PredictVehSpd3_kph]  "VVMC_PredictVehSpd3_kph"
  Add2/1 -> Relational Operator1/1
  Constant4/1 -> Relational Operator1/2
  Relational Operator1/1 -> Switch1/2
  Max3/1 -> [VVMC_Min4WhlPreVehSpd_kph]  "VVMC_Min4WhlPreVehSpd_kph"
  [VVMC_LFPreVehSpd_kph] -> Max3/1
  [VVMC_RFPreVehSpd_kph] -> Max3/2
  [VVMC_LRPreVehSpd_kph] -> Max3/3
  [VVMC_RRPreVehSpd_kph] -> Max3/4
  Max2/1 -> [VVMC_Max4WhlPreVehSpd_kph]  "VVMC_Max4WhlPreVehSpd_kph"
  [VVMC_RRPreVehSpd_kph] -> Max2/4
  [VVMC_LRPreVehSpd_kph] -> Max2/3
  [VVMC_RFPreVehSpd_kph] -> Max2/2
  [VVMC_LFPreVehSpd_kph] -> Max2/1
  Divide/1 -> [VVMC_PredictVehSpd2_kph]  "VVMC_PredictVehSpd2_kph"
  Constant3/1 -> Divide/2
  Add1/1 -> Divide/1
  [VVMC_RRPreVehSpd_kph] -> Add1/4
  [VVMC_LRPreVehSpd_kph] -> Add1/3
  [VVMC_RFPreVehSpd_kph] -> Add1/2
  [VVMC_LFPreVehSpd_kph] -> Add1/1
  VVMC_RRPreVehSpd_kph/1 -> [VVMC_RRPreVehSpd_kph]
  VVMC_LRPreVehSpd_kph/1 -> [VVMC_LRPreVehSpd_kph]
  VVMC_RFPreVehSpd_kph/1 -> [VVMC_RFPreVehSpd_kph]
  VVMC_LFPreVehSpd_kph/1 -> [VVMC_LFPreVehSpd_kph]
  VTQD_AfterAvailableTqDemRr_Nm/1 -> [VTQD_AfterAvailableTqDemRr_Nm]
  VTQD_AfterAvailableTqDemFr_Nm/1 -> [VTQD_AfterAvailableTqDemFr_Nm]
  VVMC_RR4WhlSpdSlideRate_pct/1 -> [VVMC_RR4WhlSpdSlideRate_pct]
  VVMC_LR4WhlSpdSlideRate_pct/1 -> [VVMC_LR4WhlSpdSlideRate_pct]
  VVMC_RF4WhlSpdSlideRate_pct/1 -> [VVMC_RF4WhlSpdSlideRate_pct]
  VVMC_LF4WhlSpdSlideRate_pct/1 -> [VVMC_LF4WhlSpdSlideRate_pct]
  VVMC_RRWhlSkid_flg/1 -> [VVMC_RRWhlSkid_flg]
  VVMC_LRWhlSkid_flg/1 -> [VVMC_LRWhlSkid_flg]
  VVMC_RFWhlSkid_flg/1 -> [VVMC_RFWhlSkid_flg]
  VVMC_LFWhlSkid_flg/1 -> [VVMC_LFWhlSkid_flg]
  [VVMC_4WhlSpdSlideRate_pct] -> VVMC_4WhlSpdSlideRate_pct/1
  [VVMC_AllWhlSkid_flg] -> VVMC_AllWhlSkid_flg/1
  [VVMC_PredictVehSpd_kph] -> VVMC_PredictVehSpd_kph/1
  VTQD_GearActualPosn_enum/1 -> [VTQD_GearActualPosn_enum]
  VVMC_4WheelLongAcc_Gps/1 -> [VVMC_4WheelLongAcc_Gps]
  task_time_s/1 -> [task_time_s]
  VVMC_VehicleSpeed_kph/1 -> [VVMC_VehicleSpeed_kph]
  [VVMC_LR4WhlSpdSlideRate_pct] -> Max1/3
  Constant48/1 -> OR1/2
  Constant44/1 -> Product3/2
  Max/1 -> [VVMC_Max4WhlSpdSlideRate_pct]  "VVMC_Max4WhlSpdSlideRate_pct"
  Add17/1 -> Relational Operator16/1
  Constant47/1 -> Equal1/2
  [VVMC_Min4WhlSpdSlideRate_pct] -> Switch9/1
  Equal1/1 -> OR/2
  [VVMC_RF4WhlSpdSlideRate_pct] -> Max1/2
  Delay/1 -> Product/1
  Constant46/1 -> Equal/2
  Product1/1 -> Add/1  "VVMC_DeltaVehSpd_mps"
  OR1/1 -> Switch/2
  [VTQD_AfterAvailableTqDemFr_Nm] -> Add17/1
  [VVMC_RR4WhlSpdSlideRate_pct] -> Max1/4
  [VTQD_GearActualPosn_enum] -> Equal/1
  Saturation/1 -> Add/2
  Max1/1 -> [VVMC_Min4WhlSpdSlideRate_pct]  "VVMC_Min4WhlSpdSlideRate_pct"
  [VVMC_Max4WhlSpdSlideRate_pct] -> Switch9/3
  [VVMC_RFWhlSkid_flg] -> AND/2
  [VVMC_LF4WhlSpdSlideRate_pct] -> Max/1
  [VTQD_AfterAvailableTqDemRr_Nm] -> Add17/2
  [VVMC_LF4WhlSpdSlideRate_pct] -> Max1/1
  [VVMC_4WheelLongAcc_Gps] -> Product1/1
  [VVMC_LR4WhlSpdSlideRate_pct] -> Max/3
  Delay5/1 -> Product3/1
  Product3/1 -> Switch/1
  Product/1 -> Switch/3
  Switch/1 -> Saturation/1  "VVMC_LastPredictVehSpd_mps"
  OR/1 -> Switch10/2
  [VVMC_RR4WhlSpdSlideRate_pct] -> Max/4
  [VVMC_AllWhlSkid_flg] -> OR1/1
  [task_time_s] -> Product1/3
  [VVMC_VehicleSpeed_kph] -> Delay/1
  [VVMC_RF4WhlSpdSlideRate_pct] -> Max/2
  [VVMC_VehicleSpeed_kph] -> Switch10/3
  Constant1/1 -> Product1/2
  Switch10/1 -> [VVMC_PredictVehSpd1_kph]  "VVMC_PredictVehSpd1_kph"
  AND/1 -> [VVMC_AllWhlSkid_flg]  "VVMC_AllWhlSkid_flg"
  Equal/1 -> OR/1
  Constant2/1 -> Product2/2
  [VTQD_GearActualPosn_enum] -> Equal1/1
  [VVMC_LFWhlSkid_flg] -> AND/1
  Constant11/1 -> Product/2
  Switch9/1 -> [VVMC_4WhlSpdSlideRate_pct]  "VVMC_4WhlSpdSlideRate_pct"
  Constant45/1 -> Relational Operator16/2
  [VVMC_LRWhlSkid_flg] -> AND/3
  Relational Operator16/1 -> Switch9/2
  Product2/1 -> Switch10/1
  Add/1 -> Product2/1  "VVMC_CalPredictVehSpd_mps"
  [VVMC_RRWhlSkid_flg] -> AND/4

== system vmc/VMC/VMC/Slide Rate  Calculation/4Wheel Calculation/LF Wheel ==
  VVMC_4WheelLongAcc_Gps : Inport
  task_time_s : Inport  Port=2
  VINP_LFRawWhlSpeed_kph : Inport  Port=3
  VTQD_GearActualPosn_enum : Inport  Port=4
  AND1 : Logic  Inputs=3  AllPortsSameDT=off  OutDataTypeStr=boolean
  Abs : Abs
  Add : Sum
  Add{1,5,9..10} (4 alike) : Sum  Inputs=+-
  Constant1 : Constant  Value=GRAVITY_G
  Constant11 : Constant  Value=KPH2MPS
  Constant2 : Constant  Value=MPS2KPH
  Constant24 : Constant  Value=KPH2MPS
  Constant25 : Constant  Value=GRAVITY_G
  Constant26 : Constant  Value=KVMC_WhlSpdCalAccTs_c
  Constant3 : Constant  Value=KVMC_4WheelEnSkidDetSpd_kph
  Constant36 : Constant  Value=KVMC_WheelSkidAccDev_Gps
  Constant37 : Constant  Value=KVMC_SkidRecVehSpdDev_kph
  Constant44 : Constant  Value=KPH2MPS
  Constant46 : Constant  Value=ENUM_GEARACTUALPOSN_D
  Constant47 : Constant  Value=ENUM_GEARACTUALPOSN_R
  Constant48 : Constant  Value=KVMC_PreVehSpdCalSW_flg
  Constant5 : Constant  Value=KVMC_RawWhlSpeedDeadZone_kph
  Constant52 : Constant  Value=KVMC_LFWhlSkidReset_flg
  Constant6 : Constant  Value=ONE_FLOAT
  Constant7 : Constant  Value=ONE_PERCENT
  Constant8 : Constant  Value=KVMC_RawWhlSpeedDeadZone_kph
  Constant9 : Constant  Value=ZERO_FLOAT
  Delay{,1,5..7,14} (6 alike) : Delay  DelayLength=1
  Divide : Product  Inputs=**//
  Divide1 : Product  Inputs=*//
  Equal : RelationalOperator  Operator===  OutDataTypeStr=boolean  RndMeth=Simplest
  Equal1 : RelationalOperator  Operator===  OutDataTypeStr=boolean  RndMeth=Simplest
  FirstOrderFilter : hcu_lib/Basic_Blocks/FirstOrderFilter
  OR : Logic  Operator=OR  AllPortsSameDT=off  OutDataTypeStr=boolean
  OR1 : Logic  Operator=OR  AllPortsSameDT=off  OutDataTypeStr=boolean
  OR2 : Logic  Operator=OR  AllPortsSameDT=off  OutDataTypeStr=boolean
  Product : Product
  Product1 : Product  Inputs=3
  Product2 : Product
  Product3 : Product
  Relational Operator : RelationalOperator  Operator=>  OutDataTypeStr=boolean  RndMeth=Simplest
  Relational Operator{1..3,9} (4 alike) : RelationalOperator  Operator=<=  OutDataTypeStr=boolean  RndMeth=Simplest
  SR_Latch : hcu_lib/Basic_Blocks/SR_Latch
  Saturation : Saturate  UpperLimit=KVMC_PredVehSpdLimit_mps  LowerLimit=ZERO_FLOAT
  Switch{,2..3,10} (4 alike) : Switch  Criteria=u2 > Threshold
  VVMC_LFPreVehSpd_kph : Outport
  VVMC_LFWhlSkid_flg : Outport  Port=2
  VVMC_LF4WhlSpdSlideRate_pct : Outport  Port=3
  wires:
  [VINP_LFRawWhlSpeed_kph] -> Relational Operator1/1
  Constant3/1 -> Relational Operator1/2
  Relational Operator1/1 -> OR2/1
  AND1/1 -> OR2/2
  OR2/1 -> SR_Latch/2  "VVMC_LFWhlSkidReset_flg"
  [VVMC_LF4WhlSpdSlideRate_pct] -> VVMC_LF4WhlSpdSlideRate_pct/1
  [VVMC_LFWhlSkid_flg] -> VVMC_LFWhlSkid_flg/1
  [VVMC_LFPreVehSpd_kph] -> VVMC_LFPreVehSpd_kph/1
  VTQD_GearActualPosn_enum/1 -> [VTQD_GearActualPosn_enum]
  [VVMC_LFWhlSkid_flg] -> OR1/1
  VINP_LFRawWhlSpeed_kph/1 -> [VINP_LFRawWhlSpeed_kph]
  task_time_s/1 -> [task_time_s]
  VVMC_4WheelLongAcc_Gps/1 -> [VVMC_4WheelLongAcc_Gps]
  [VVMC_LFPreVehSpd_kph] -> Delay6/1
  [VINP_LFRawWhlSpeed_kph] -> Delay/1
  [VVMC_LFPreVehSpd_kph] -> Delay5/1
  Add/1 -> Product2/1  "VVMC_LFCalPreVehSpd_mps"
  [task_time_s] -> Product1/3
  Constant11/1 -> Product/2
  Constant1/1 -> Product1/2
  Equal/1 -> OR/1
  Constant2/1 -> Product2/2
  Switch/1 -> Saturation/1  "VVMC_LFLastPreVehSpd_mps"
  Product/1 -> Switch/3
  Delay5/1 -> Product3/1
  Product3/1 -> Switch/1
  [VVMC_4WheelLongAcc_Gps] -> Product1/1
  OR/1 -> Switch10/2
  [VTQD_GearActualPosn_enum] -> Equal/1
  [VINP_LFRawWhlSpeed_kph] -> Switch10/3
  Delay/1 -> Product/1
  [VTQD_GearActualPosn_enum] -> Equal1/1
  Saturation/1 -> Add/2
  Product1/1 -> Add/1  "VVMC_LFDeltaVehSpd_mps"
  Constant46/1 -> Equal/2
  Equal1/1 -> OR/2
  OR1/1 -> Switch/2
  Product2/1 -> Switch10/1
  Constant47/1 -> Equal1/2
  Switch10/1 -> [VVMC_LFPreVehSpd_kph]  "VVMC_LFPreVehSpd_kph"
  Constant44/1 -> Product3/2
  Constant48/1 -> OR1/2
  FirstOrderFilter/1 -> [VVMC_LFWhlCalAcc_Gps]  "VVMC_LFWhlCalAcc_Gps"
  Add5/1 -> Divide/1
  [VINP_LFRawWhlSpeed_kph] -> Delay1/1
  Constant24/1 -> Divide/2
  Constant25/1 -> Divide/4
  [task_time_s] -> Divide/3
  [VINP_LFRawWhlSpeed_kph] -> Relational Operator3/1
  Delay1/1 -> Add5/2
  [VINP_LFRawWhlSpeed_kph] -> Add1/1
  [VVMC_LFPreVehSpd_kph] -> Switch2/3
  Constant7/1 -> Divide1/2
  Delay7/1 -> Add10/2
  Add1/1 -> Divide1/1
  Relational Operator/1 -> SR_Latch/1
  Switch3/1 -> [VVMC_LF4WhlSpdSlideRate_pct]  "VVMC_LF4WhlSpdSlideRate_pct"
  Add9/1 -> Relational Operator/1
  Constant5/1 -> Relational Operator2/2
  [VVMC_LFPreVehSpd_kph] -> Relational Operator2/1
  [VVMC_LFWhlCalAcc_Gps] -> Add9/1
  Divide/1 -> FirstOrderFilter/1
  Relational Operator2/1 -> Switch2/2
  Switch2/1 -> Divide1/3
  [VVMC_LFPreVehSpd_kph] -> Add1/2
  [VINP_LFRawWhlSpeed_kph] -> Add5/1
  Divide1/1 -> Switch3/3  "VVMC_LFCal4WhlSpdSlideRate_pct"
  SR_Latch/1 -> [VVMC_LFWhlSkid_flg]  "VVMC_LFWhlSkid_flg"
  Delay6/1 -> Add10/1
  Constant26/1 -> FirstOrderFilter/3
  [task_time_s] -> FirstOrderFilter/2
  Add10/1 -> Abs/1
  Relational Operator3/1 -> Switch3/2
  [VVMC_LFWhlSkid_flg] -> Delay14/1
  [VVMC_4WheelLongAcc_Gps] -> Add9/2
  Abs/1 -> Relational Operator9/1
  Delay14/1 -> AND1/2
  Constant6/1 -> Switch2/1
  Constant8/1 -> Relational Operator3/2
  Constant52/1 -> AND1/3
  Constant36/1 -> Relational Operator/2
  Constant9/1 -> Switch3/1
  Relational Operator9/1 -> AND1/1
  Constant37/1 -> Relational Operator9/2
  [VINP_LFRawWhlSpeed_kph] -> Delay7/1

== system vmc/VMC/VMC/Slide Rate  Calculation/4Wheel Calculation/LR Wheel ==
  VVMC_4WheelLongAcc_Gps : Inport
  task_time_s : Inport  Port=2
  VINP_LRRawWhlSpeed_kph : Inport  Port=3
  VTQD_GearActualPosn_enum : Inport  Port=4
  AND3 : Logic  Inputs=3  AllPortsSameDT=off  OutDataTypeStr=boolean
  Abs2 : Abs
  Add : Sum
  Add{4,7,13..14} (4 alike) : Sum  Inputs=+-
  Constant1 : Constant  Value=GRAVITY_G
  Constant11 : Constant  Value=KPH2MPS
  Constant19 : Constant  Value=ONE_PERCENT
  Constant2 : Constant  Value=MPS2KPH
  Constant20 : Constant  Value=KVMC_RawWhlSpeedDeadZone_kph
  Constant21 : Constant  Value=ZERO_FLOAT
  Constant22 : Constant  Value=KVMC_RawWhlSpeedDeadZone_kph
  Constant23 : Constant  Value=ONE_FLOAT
  Constant30 : Constant  Value=KPH2MPS
  Constant31 : Constant  Value=GRAVITY_G
  Constant32 : Constant  Value=KVMC_WhlSpdCalAccTs_c
  Constant40 : Constant  Value=KVMC_WheelSkidAccDev_Gps
  Constant41 : Constant  Value=KVMC_SkidRecVehSpdDev_kph
  Constant44 : Constant  Value=KPH2MPS
  Constant46 : Constant  Value=ENUM_GEARACTUALPOSN_D
  Constant47 : Constant  Value=ENUM_GEARACTUALPOSN_R
  Constant48 : Constant  Value=KVMC_PreVehSpdCalSW_flg
  Constant5 : Constant  Value=KVMC_4WheelEnSkidDetSpd_kph
  Constant50 : Constant  Value=KVMC_LRWhlSkidReset_flg
  Delay{,3,5,10..11,16} (6 alike) : Delay  DelayLength=1
  Divide4 : Product  Inputs=*//
  Divide6 : Product  Inputs=**//
  Equal : RelationalOperator  Operator===  OutDataTypeStr=boolean  RndMeth=Simplest
  Equal1 : RelationalOperator  Operator===  OutDataTypeStr=boolean  RndMeth=Simplest
  FirstOrderFilter2 : hcu_lib/Basic_Blocks/FirstOrderFilter
  OR : Logic  Operator=OR  AllPortsSameDT=off  OutDataTypeStr=boolean
  OR1 : Logic  Operator=OR  AllPortsSameDT=off  OutDataTypeStr=boolean
  OR2 : Logic  Operator=OR  AllPortsSameDT=off  OutDataTypeStr=boolean
  Product : Product
  Product1 : Product  Inputs=3
  Product2 : Product
  Product3 : Product
  Relational Operator12 : RelationalOperator  Operator=>  OutDataTypeStr=boolean  RndMeth=Simplest
  Relational Operator{2,7..8,13} (4 alike) : RelationalOperator  Operator=<=  OutDataTypeStr=boolean  RndMeth=Simplest
  SR_Latch2 : hcu_lib/Basic_Blocks/SR_Latch
  Saturation : Saturate  UpperLimit=KVMC_PredVehSpdLimit_mps  LowerLimit=ZERO_FLOAT
  Switch{,7..8,10} (4 alike) : Switch  Criteria=u2 > Threshold
  VVMC_LRPreVehSpd_kph : Outport
  VVMC_LRWhlSkid_flg : Outport  Port=2
  VVMC_LR4WhlSpdSlideRate_pct : Outport  Port=3
  wires:
  OR2/1 -> SR_Latch2/2  "VVMC_LRWhlSkidReset_flg"
  AND3/1 -> OR2/2
  Constant5/1 -> Relational Operator2/2
  Relational Operator2/1 -> OR2/1
  [VINP_LRRawWhlSpeed_kph] -> Relational Operator2/1
  [VVMC_LR4WhlSpdSlideRate_pct] -> VVMC_LR4WhlSpdSlideRate_pct/1
  [VVMC_LRWhlSkid_flg] -> VVMC_LRWhlSkid_flg/1
  [VVMC_LRPreVehSpd_kph] -> VVMC_LRPreVehSpd_kph/1
  VTQD_GearActualPosn_enum/1 -> [VTQD_GearActualPosn_enum]
  VINP_LRRawWhlSpeed_kph/1 -> [VINP_LRRawWhlSpeed_kph]
  VVMC_4WheelLongAcc_Gps/1 -> [VVMC_4WheelLongAcc_Gps]
  task_time_s/1 -> [task_time_s]
  Relational Operator8/1 -> Switch8/2
  Add4/1 -> Divide4/1
  [VVMC_LRPreVehSpd_kph] -> Switch7/3
  Switch7/1 -> Divide4/3
  Divide4/1 -> Switch8/3  "VVMC_LRCal4WhlSpdSlideRate_pct"
  Constant21/1 -> Switch8/1
  Constant20/1 -> Relational Operator8/2
  [VVMC_LRPreVehSpd_kph] -> Add4/2
  Constant23/1 -> Switch7/1
  Switch8/1 -> [VVMC_LR4WhlSpdSlideRate_pct]  "VVMC_LR4WhlSpdSlideRate_pct"
  Constant19/1 -> Divide4/2
  [VVMC_LRPreVehSpd_kph] -> Relational Operator7/1
  Relational Operator7/1 -> Switch7/2
  [VINP_LRRawWhlSpeed_kph] -> Relational Operator8/1
  [VINP_LRRawWhlSpeed_kph] -> Add4/1
  Constant22/1 -> Relational Operator7/2
  [VVMC_LRPreVehSpd_kph] -> Delay10/1
  [VVMC_LRWhlSkid_flg] -> OR1/1
  OR/1 -> Switch10/2
  Saturation/1 -> Add/2
  Delay5/1 -> Product3/1
  Product/1 -> Switch/3
  Delay/1 -> Product/1
  Product1/1 -> Add/1  "VVMC_LRDeltaVehSpd_mps"
  Constant2/1 -> Product2/2
  Constant46/1 -> Equal/2
  [VTQD_GearActualPosn_enum] -> Equal1/1
  Equal1/1 -> OR/2
  Constant47/1 -> Equal1/2
  Constant48/1 -> OR1/2
  OR1/1 -> Switch/2
  [VINP_LRRawWhlSpeed_kph] -> Delay/1
  Switch10/1 -> [VVMC_LRPreVehSpd_kph]  "VVMC_LRPreVehSpd_kph"
  Product3/1 -> Switch/1
  Constant1/1 -> Product1/2
  [VINP_LRRawWhlSpeed_kph] -> Switch10/3
  [VTQD_GearActualPosn_enum] -> Equal/1
  Equal/1 -> OR/1
  Add/1 -> Product2/1  "VVMC_LRCalPreVehSpd_mps"
  Constant11/1 -> Product/2
  Product2/1 -> Switch10/1
  Switch/1 -> Saturation/1  "VVMC_LRLastPreVehSpd_mps"
  Constant44/1 -> Product3/2
  [VVMC_4WheelLongAcc_Gps] -> Product1/1
  [task_time_s] -> Product1/3
  [VVMC_LRPreVehSpd_kph] -> Delay5/1
  [task_time_s] -> FirstOrderFilter2/2
  Add14/1 -> Relational Operator12/1
  Add13/1 -> Abs2/1
  Constant40/1 -> Relational Operator12/2
  [VVMC_4WheelLongAcc_Gps] -> Add14/2
  Divide6/1 -> FirstOrderFilter2/1
  FirstOrderFilter2/1 -> [VVMC_LRWhlCalAcc_Gps]  "VVMC_LRWhlCalAcc_Gps"
  Constant32/1 -> FirstOrderFilter2/3
  [VVMC_LRWhlCalAcc_Gps] -> Add14/1
  [VINP_LRRawWhlSpeed_kph] -> Delay3/1
  [VINP_LRRawWhlSpeed_kph] -> Add7/1
  Delay11/1 -> Add13/2
  Relational Operator12/1 -> SR_Latch2/1
  Add7/1 -> Divide6/1
  Delay16/1 -> AND3/2
  Abs2/1 -> Relational Operator13/1
  Relational Operator13/1 -> AND3/1
  [VVMC_LRWhlSkid_flg] -> Delay16/1
  SR_Latch2/1 -> [VVMC_LRWhlSkid_flg]  "VVMC_LRWhlSkid_flg"
  [VINP_LRRawWhlSpeed_kph] -> Delay11/1
  Constant31/1 -> Divide6/4
  Constant50/1 -> AND3/3
  Constant41/1 -> Relational Operator13/2
  [task_time_s] -> Divide6/3
  Constant30/1 -> Divide6/2
  Delay10/1 -> Add13/1
  Delay3/1 -> Add7/2

== system vmc/VMC/VMC/Slide Rate  Calculation/4Wheel Calculation/RF Wheel ==
  VVMC_4WheelLongAcc_Gps : Inport
  task_time_s : Inport  Port=2
  VINP_RFRawWhlSpeed_kph : Inport  Port=3
  VTQD_GearActualPosn_enum : Inport  Port=4
  AND2 : Logic  Inputs=3  AllPortsSameDT=off  OutDataTypeStr=boolean
  Abs1 : Abs
  Add : Sum
  Add{2,6,11..12} (4 alike) : Sum  Inputs=+-
  Constant1 : Constant  Value=GRAVITY_G
  Constant10 : Constant  Value=ONE_PERCENT
  Constant11 : Constant  Value=KPH2MPS
  Constant12 : Constant  Value=KVMC_RawWhlSpeedDeadZone_kph
  Constant13 : Constant  Value=ZERO_FLOAT
  Constant2 : Constant  Value=MPS2KPH
  Constant27 : Constant  Value=KPH2MPS
  Constant28 : Constant  Value=GRAVITY_G
  Constant29 : Constant  Value=KVMC_WhlSpdCalAccTs_c
  Constant3 : Constant  Value=KVMC_RawWhlSpeedDeadZone_kph
  Constant38 : Constant  Value=KVMC_WheelSkidAccDev_Gps
  Constant39 : Constant  Value=KVMC_SkidRecVehSpdDev_kph
  Constant4 : Constant  Value=ONE_FLOAT
  Constant44 : Constant  Value=KPH2MPS
  Constant46 : Constant  Value=ENUM_GEARACTUALPOSN_D
  Constant47 : Constant  Value=ENUM_GEARACTUALPOSN_R
  Constant48 : Constant  Value=KVMC_PreVehSpdCalSW_flg
  Constant5 : Constant  Value=KVMC_4WheelEnSkidDetSpd_kph
  Constant51 : Constant  Value=KVMC_RFWhlSkidReset_flg
  Delay{,2,5,8..9,15} (6 alike) : Delay  DelayLength=1
  Divide2 : Product  Inputs=*//
  Divide5 : Product  Inputs=**//
  Equal : RelationalOperator  Operator===  OutDataTypeStr=boolean  RndMeth=Simplest
  Equal1 : RelationalOperator  Operator===  OutDataTypeStr=boolean  RndMeth=Simplest
  FirstOrderFilter1 : hcu_lib/Basic_Blocks/FirstOrderFilter
  OR : Logic  Operator=OR  AllPortsSameDT=off  OutDataTypeStr=boolean
  OR1 : Logic  Operator=OR  AllPortsSameDT=off  OutDataTypeStr=boolean
  OR2 : Logic  Operator=OR  AllPortsSameDT=off  OutDataTypeStr=boolean
  Product : Product
  Product1 : Product  Inputs=3
  Product2 : Product
  Product3 : Product
  Relational Operator{1..2,4,11} (4 alike) : RelationalOperator  Operator=<=  OutDataTypeStr=boolean  RndMeth=Simplest
  Relational Operator10 : RelationalOperator  Operator=>  OutDataTypeStr=boolean  RndMeth=Simplest
  SR_Latch1 : hcu_lib/Basic_Blocks/SR_Latch
  Saturation : Saturate  UpperLimit=KVMC_PredVehSpdLimit_mps  LowerLimit=ZERO_FLOAT
  Switch{,1,4,10} (4 alike) : Switch  Criteria=u2 > Threshold
  VVMC_RFPreVehSpd_kph : Outport
  VVMC_RFWhlSkid_flg : Outport  Port=2
  VVMC_RF4WhlSpdSlideRate_pct : Outport  Port=3
  wires:
  OR2/1 -> SR_Latch1/2  "VVMC_RFWhlSkidReset_flg"
  AND2/1 -> OR2/2
  [VINP_RFRawWhlSpeed_kph] -> Relational Operator2/1
  Relational Operator2/1 -> OR2/1
  Constant5/1 -> Relational Operator2/2
  [VVMC_RF4WhlSpdSlideRate_pct] -> VVMC_RF4WhlSpdSlideRate_pct/1
  [VVMC_RFWhlSkid_flg] -> VVMC_RFWhlSkid_flg/1
  [VVMC_RFPreVehSpd_kph] -> VVMC_RFPreVehSpd_kph/1
  task_time_s/1 -> [task_time_s]
  VVMC_4WheelLongAcc_Gps/1 -> [VVMC_4WheelLongAcc_Gps]
  VINP_RFRawWhlSpeed_kph/1 -> [VINP_RFRawWhlSpeed_kph]
  VTQD_GearActualPosn_enum/1 -> [VTQD_GearActualPosn_enum]
  [VVMC_RFPreVehSpd_kph] -> Switch1/3
  [VVMC_RFPreVehSpd_kph] -> Relational Operator1/1
  [VVMC_RFPreVehSpd_kph] -> Add2/2
  [VVMC_RFPreVehSpd_kph] -> Delay8/1
  [VVMC_RFWhlSkid_flg] -> OR1/1
  Add/1 -> Product2/1  "VVMC_RFCalPreVehSpd_mps"
  Equal/1 -> OR/1
  [task_time_s] -> Product1/3
  [VVMC_4WheelLongAcc_Gps] -> Product1/1
  Constant44/1 -> Product3/2
  Switch/1 -> Saturation/1  "VVMC_RFLastPreVehSpd_mps"
  Constant11/1 -> Product/2
  Product2/1 -> Switch10/1
  Constant1/1 -> Product1/2
  Switch10/1 -> [VVMC_RFPreVehSpd_kph]  "VVMC_RFPreVehSpd_kph"
  Constant48/1 -> OR1/2
  Constant47/1 -> Equal1/2
  OR1/1 -> Switch/2
  Constant46/1 -> Equal/2
  Equal1/1 -> OR/2
  Product1/1 -> Add/1  "VVMC_RFDeltaVehSpd_mps"
  Constant2/1 -> Product2/2
  Saturation/1 -> Add/2
  Delay/1 -> Product/1
  [VTQD_GearActualPosn_enum] -> Equal1/1
  [VINP_RFRawWhlSpeed_kph] -> Switch10/3
  [VTQD_GearActualPosn_enum] -> Equal/1
  OR/1 -> Switch10/2
  [VINP_RFRawWhlSpeed_kph] -> Delay/1
  [VVMC_RFPreVehSpd_kph] -> Delay5/1
  Product3/1 -> Switch/1
  Delay5/1 -> Product3/1
  Product/1 -> Switch/3
  [task_time_s] -> Divide5/3
  Delay2/1 -> Add6/2
  Add2/1 -> Divide2/1
  Switch4/1 -> [VVMC_RF4WhlSpdSlideRate_pct]  "VVMC_RF4WhlSpdSlideRate_pct"
  FirstOrderFilter1/1 -> [VVMC_RFWhlCalAcc_Gps]  "VVMC_RFWhlCalAcc_Gps"
  Constant29/1 -> FirstOrderFilter1/3
  [VVMC_RFWhlCalAcc_Gps] -> Add12/1
  SR_Latch1/1 -> [VVMC_RFWhlSkid_flg]  "VVMC_RFWhlSkid_flg"
  Relational Operator10/1 -> SR_Latch1/1
  [VINP_RFRawWhlSpeed_kph] -> Relational Operator4/1
  [VINP_RFRawWhlSpeed_kph] -> Add2/1
  Constant10/1 -> Divide2/2
  Add6/1 -> Divide5/1
  Constant51/1 -> AND2/3
  Relational Operator4/1 -> Switch4/2
  Constant4/1 -> Switch1/1
  Constant39/1 -> Relational Operator11/2
  Delay9/1 -> Add11/2
  [task_time_s] -> FirstOrderFilter1/2
  Abs1/1 -> Relational Operator11/1
  [VINP_RFRawWhlSpeed_kph] -> Delay9/1
  Delay8/1 -> Add11/1
  Divide2/1 -> Switch4/3  "VVMC_RFCal4WhlSpdSlideRate_pct"
  Constant38/1 -> Relational Operator10/2
  Add11/1 -> Abs1/1
  Constant28/1 -> Divide5/4
  Relational Operator1/1 -> Switch1/2
  Constant27/1 -> Divide5/2
  [VVMC_RFWhlSkid_flg] -> Delay15/1
  Delay15/1 -> AND2/2
  Constant3/1 -> Relational Operator1/2
  [VINP_RFRawWhlSpeed_kph] -> Delay2/1
  Constant13/1 -> Switch4/1
  [VINP_RFRawWhlSpeed_kph] -> Add6/1
  Add12/1 -> Relational Operator10/1
  Constant12/1 -> Relational Operator4/2
  Divide5/1 -> FirstOrderFilter1/1
  Relational Operator11/1 -> AND2/1
  Switch1/1 -> Divide2/3
  [VVMC_4WheelLongAcc_Gps] -> Add12/2
